simulink model "mbd_example_test"  (R2022b)
settings: Solver=FixedStepDiscrete  StartTime=0.0  StopTime=10.0  RelTol=1e-3  EnableMultiTasking=on
PostLoadFcn:
  | run([bdroot '_init']);
InitFcn:
  | checkModelFolder(true); % Optional
  | run([bdroot '_init']);
undefined symbols (not defined in the file or in its folder): MBDDiag_Comm_Module, MBDDiag_Comm_Type
libraries: MbdLib_Uart x9, MbdLib_Usb x8, MbdLib_Digital x7, MbdLib_Pwm x6, MbdLib_Qdec x6, MbdLib_Sys x5, MbdLib_LpTimer x5, MbdLib_Nvmem x5, MbdLib_Analog x4, MbdLib_Can x3, MbdLib_I2c x2, MbdLib_Ic x2
settings Model: Creator=KenYoshioka  LastModifiedBy=KenYoshioka
settings SolverCC: AutoInsertRateTranBlk=on
settings OptimizationCC: DefaultParameterBehavior=Inlined  DefaultUnderspecifiedDataType=single  EnhancedBackFolding=on  BooleansAsBitfields=on  PassReuseOutputArgsAs=Individual arguments  ZeroExternalMemoryAtStartup=off  ZeroInternalMemoryAtStartup=off  OptimizeBlockOrder=speed  DifferentSizesBufferReuse=on  EfficientTunableParamExpr=on
settings DebuggingCC: ParameterTunabilityLossMsg=error
settings HardwareCC: ProdBitPerPointer=32  ProdBitPerSizeT=32  ProdBitPerPtrDiffT=32  ProdLargestAtomicInteger=Long  ProdLargestAtomicFloat=Double  ProdWordSize=32  ProdHWDeviceType=ARM Compatible->ARM Cortex-M
settings ModelReferenceCC: EnableRefExpFcnMdlSchedulingChecks=on  ModelReferenceNumInstancesAllowed=Single
settings SFSimCC: MATLABDynamicMemAlloc=off
settings RTWCC: Description=MBD Embedded Target STM32 Cortex M4 (real-time)  SystemTargetFile=MBD_STM32_stf.tlc  TemplateMakefile=MBD_STM32.tmf  Toolchain=arm-none-eabi - v9.3.1
settings CodeAppCC: ForceParamTrailComments=on  IgnoreCustomStorageClasses=off  MaxIdLength=255  OperatorAnnotations=on  SimulinkDataObjDesc=on  SFDataObjDesc=on  InsertBlockDesc=on
settings STFCustomTargetCC: MultiwordLength=256  IncludeMdlTerminateFcn=off  CombineOutputUpdateFcns=on  CombineSignalStateStructs=on  SuppressErrorStatus=on  ERTCustomFileBanners=on  SupportContinuousTime=off  RemoveResetFunc=on  MATLABClassNameForMDSCustomization=Simulink.SoftwareTarget.ERTCustomization  UseToolchainInfoCompliant=on  SystemTargetFile=MBD_STM32_stf.tlc
settings ERTTargetCC: ParMdlRefBuildCompliant=off  CompOptLevelCompliant=off  ConcurrentExecutionCompliant=off  IncludeMdlTerminateFcn=off  CombineSignalStateStructs=on  SuppressErrorStatus=on  SupportNonInlinedSFcns=on  ModelStepFunctionPrototypeControlCompliant=off  CPPClassGenCompliant=off  ExtModeStaticAllocSize=2000  InlinedParameterPlacement=NonHierarchical  ERTCustomFileTemplate=mbd_lib_interface.tlc  MaxLineWidth=110

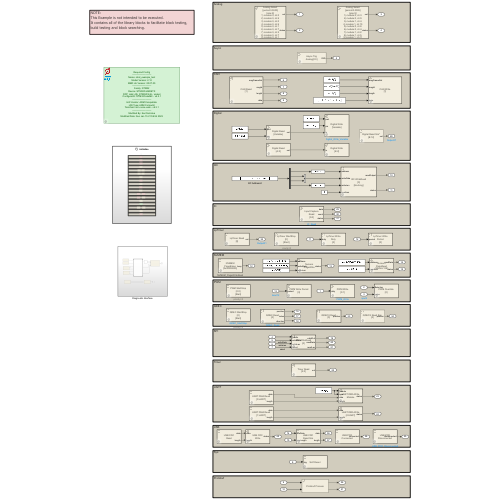
[thumbnail: Simulink's stored preview of the top-level diagram]
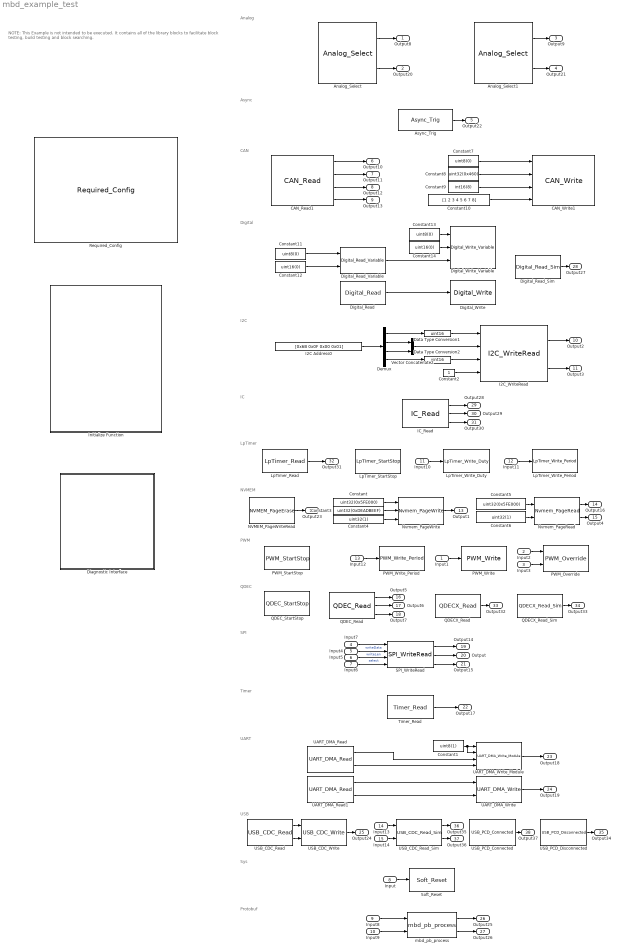
== system mbd_example_test ==
  note: NOTE:
      | This Example is not intended to be executed.
      | It contains all of the library blocks to facilitate block testing,
      | build testing and block searching.
  note: UART
  note: SPI
  note: NVMEM
  note: I2C
  note: CAN
  note: Digital
  note: QDEC
  note: PWM
  note: Analog
  note: Timer
  note: Async
  note: USB
  note: Sys
  note: Protobuf
  note: IC
  note: LpTimer
  Input1 : Inport
  Input2 : Inport  Port=2
  Input3 : Inport  Port=3
  Input7 : Inport  Port=4  OutDataTypeStr=boolean
  Input4 : Inport  Port=5  OutDataTypeStr=uint8
  Input5 : Inport  Port=6  OutDataTypeStr=uint16
  Input6 : Inport  Port=7
  Input : Inport  Port=8
  Input8 : Inport  Port=9
  Input9 : Inport  Port=10
  Input10 : Inport  Port=11
  Input11 : Inport  Port=12
  Input12 : Inport  Port=13
  Input13 : Inport  Port=14
  Input14 : Inport  Port=15
  Analog_Select : MbdLib_Analog/Analog_Select  Param_triggerMode=No trigger  Param_module=0  Param_timeout=0  Param_outputNum=9  Param_module1=0  Param_index1=0  Param_module2=0  Param_index2=1  Param_module3=0  Param_index3=2  Param_module4=0  Param_index4=3  Param_module5=0  Param_index5=4  Param_module6=0  Param_index6=5  Param_module7=0  Param_index7=6  Param_module8=0  Param_index8=7  Param_module9=0  Param_index9=8  Param_module10=0  Param_index10=9  Param_module11=0  Param_index11=10  Param_module12=0  Param_index12=11  Param_sampleTime=T_s_COMM  Param_MBDUpdate=1
      settings: SourceProductName=Peloton Interface Library
  Analog_Select1 : MbdLib_Analog/Analog_Select  Param_triggerMode=No trigger  Param_module=0  Param_timeout=0  Param_outputNum=9  Param_module1=0  Param_index1=0  Param_module2=0  Param_index2=1  Param_module3=1  Param_index3=2  Param_module4=1  Param_index4=3  Param_module5=0  Param_index5=4  Param_module6=0  Param_index6=5  Param_module7=1  Param_index7=6  Param_module8=1  Param_index8=7  Param_module9=1  Param_index9=8  Param_module10=0  Param_index10=9  Param_module11=0  Param_index11=10  Param_module12=0  Param_index12=11  Param_sampleTime=T_s_COMM  Param_MBDUpdate=1
      settings: SourceProductName=Peloton Interface Library
  Async_Trig : MbdLib_Async/Async_Trig  Param_source=Analog  Param_module=0  Param_ch=0  Param_sampleTime=-1
      settings: SourceProductName=Peloton Interface Library
  CAN_Read1 : MbdLib_Can/CAN_Read  Param_module=1  Param_sampleTime=T_s_COMM
      settings: SourceProductName=Peloton Interface Library
  CAN_Write1 : MbdLib_Can/CAN_Write  Param_module=1  Param_sampleTime=T_s_COMM
      settings: SourceProductName=Peloton Interface Library
  Constant : Constant  Value=uint32(0x5FE000)
  Constant1 : Constant  Value=uint8(1)
  Constant10 : Constant  Value=[1 2 3 4 5 6 7 8]  OutDataTypeStr=uint8
  Constant11 : Constant  Value=uint8(0)
  Constant12 : Constant  Value=uint16(0)
  Constant13 : Constant  Value=uint8(0)
  Constant14 : Constant  Value=uint16(0)
  Constant2 : Constant  OutDataTypeStr=uint16
  Constant3 : Constant  Value=uint32(0xDEADBEEF)
  Constant4 : Constant  Value=uint32(1)
  Constant5 : Constant  Value=uint32(0x5FE000)
  Constant6 : Constant  Value=uint32(1)
  Constant7 : Constant  Value=uint8(0)
  Constant8 : Constant  Value=uint32(0x460)
  Constant9 : Constant  Value=int16(8)
  Data Type Conversion1 : DataTypeConversion  OutDataTypeStr=uint16  SaturateOnIntegerOverflow=off  RndMeth=Floor
  Data Type Conversion2 : DataTypeConversion  OutDataTypeStr=uint16  SaturateOnIntegerOverflow=off  RndMeth=Floor
  Demux : Demux
  Diagnostic Interface : Subsystem
  Digital_Read : MbdLib_Digital/Digital_Read  Param_module=A  Param_ch=0  Param_sampleTime=T_s_COMM  Sim_invert=off  Sim_out=0
      settings: SourceProductName=Peloton Interface Library
  Digital_Read_Sim : MbdLib_Digital/Digital_Read_Sim  Param_module=B  Param_ch=12  Param_sampleTime=Tfast_s  Sim_invert=on  Sim_out=0  Sim_enable=on  Sim_simin=sim_knob1Button
      settings: SourceProductName=Peloton Interface Library
  Digital_Read_Variable : MbdLib_Digital/Digital_Read_Variable  Param_sampleTime=T_s_COMM  Sim_invert=off  Sim_out=0
      settings: SourceProductName=Peloton Interface Library
  Digital_Write : MbdLib_Digital/Digital_Write  Param_module=E  Param_ch=2  Param_sampleTime=-1
      settings: SourceProductName=Peloton Interface Library
  Digital_Write_Variable : MbdLib_Digital/Digital_Write_Variable  Param_sampleTime=-1
      settings: SourceProductName=Peloton Interface Library
  I2C Address0 : Constant  Value=[0x6B 0x0F 0x00 0x01]  OutDataTypeStr=uint8
  I2C_WriteRead : MbdLib_I2c/I2C_WriteRead  Param_module=0  Param_writeLim=2  Param_readLim=1  Param_mode=blocking  Param_timeout=0  Param_sampleTime=T_s_COMM
      settings: SourceProductName=Peloton Interface Library
  IC_Read : MbdLib_Ic/IC_Read  Param_module=0  Param_ch=0  Param_width=byte  Param_length=0  Param_sampleTime=-1
      settings: SourceProductName=Peloton Interface Library
  Initialize Function : Subsystem  TreatAsAtomicUnit=on
  LpTimer_Read : MbdLib_LpTimer/LpTimer_Read  Param_module=0  Param_sampleTime=-1
      settings: SourceProductName=Peloton Interface Library
  LpTimer_StartStop : MbdLib_LpTimer/LpTimer_StartStop  Priority=0  Param_module=0  Param_action=Start  Param_mode=PWM  Param_period=0  Param_duty=0  Param_priority=0  Param_sampleTime=-1
      settings: AttributesFormatString=priority=%<priority>  SourceProductName=Peloton Interface Library
  LpTimer_Write_Duty : MbdLib_LpTimer/LpTimer_Write_Duty  Param_module=0  Param_sampleTime=-1
      settings: SourceProductName=Peloton Interface Library
  LpTimer_Write_Period : MbdLib_LpTimer/LpTimer_Write_Period  Param_module=0  Param_sampleTime=-1
      settings: SourceProductName=Peloton Interface Library
  NVMEM_PageWriteRead : MbdLib_Nvmem/NVMEM_PageErase  Param_address=0  Param_sampleTime=-1
      settings: SourceProductName=Peloton Interface Library
  Nvmem_PageRead : MbdLib_Nvmem/Nvmem_PageRead  Param_wordLim=128  Param_sampleTime=T_s_COMM
      settings: SourceProductName=Peloton Interface Library
  Nvmem_PageWrite : MbdLib_Nvmem/Nvmem_PageWrite  Param_sampleTime=T_s_COMM
      settings: SourceProductName=Peloton Interface Library
  PWM_Override : MbdLib_Pwm/PWM_Override  Param_module=0  Param_sampleTime=T_s_COMM
      settings: SourceProductName=Peloton Interface Library
  PWM_StartStop : MbdLib_Pwm/PWM_StartStop  Priority=0  Param_module=0  Param_ch=0  Param_action=Start  Param_priority=0  Param_sampleTime=-1
      settings: AttributesFormatString=priority=%<priority>  SourceProductName=Peloton Interface Library
  PWM_Write : MbdLib_Pwm/PWM_Write  Priority=1  Param_module=0  Param_ch_visible=1  Param_ch=1  Param_sync=off  Param_sampleTime=T_s_COMM
      settings: SourceProductName=Peloton Interface Library
  PWM_Write_Period : MbdLib_Pwm/PWM_Write_Period  Param_module=0  Param_sampleTime=-1
      settings: SourceProductName=Peloton Interface Library
  QDECX_Read : MbdLib_Qdec/QDECX_Read  Param_module=0  Param_sampleTime=-1  Sim_position=0
      settings: SourceProductName=Peloton Interface Library
  QDECX_Read_Sim : MbdLib_Qdec/QDECX_Read_Sim  Param_module=0  Param_sampleTime=-1  Sim_position=0  Sim_enable=off  Sim_simin=mbdSim_knob1Position
      settings: SourceProductName=Peloton Interface Library
  QDEC_Read : MbdLib_Qdec/QDEC_Read  Param_module=0  Param_dirOut=off  Param_sampleTime=T_s_COMM  Sim_position=0  Sim_index=0  Sim_direction=0
      settings: SourceProductName=Peloton Interface Library
  QDEC_StartStop : MbdLib_Qdec/QDEC_StartStop  Priority=0  Param_module=0  Param_action=Start  Param_priority=0  Param_sampleTime=-1
      settings: AttributesFormatString=priority=%<priority>  SourceProductName=Peloton Interface Library
  Required_Config : MbdLib_Required/Required_Config  Tag=MBD_Target_Info  Param_update=1
      settings: SourceProductName=Peloton Interface Library
  SPI_WriteRead : MbdLib_Spi/SPI_WriteRead  Param_module=0  Param_sampleTime=T_s_COMM
      settings: SourceProductName=Peloton Interface Library
  Soft_Reset : MbdLib_Sys/Soft_Reset  Param_sampleTime=-1
      settings: SourceProductName=Peloton Interface Library
  Timer_Read : MbdLib_Timer/Timer_Read  Param_module=2  Param_ch=0  Param_sampleTime=T_s_COMM
      settings: SourceProductName=Peloton Interface Library
  UART_DMA_Read : MbdLib_Uart/UART_DMA_Read  Param_module=0  Param_type=UART  Param_readLim=1  Param_sampleTime=T_s_COMM
      settings: SourceProductName=Peloton Interface Library
  UART_DMA_Read1 : MbdLib_Uart/UART_DMA_Read  Param_module=1  Param_type=UART  Param_readLim=1  Param_sampleTime=T_s_COMM
      settings: SourceProductName=Peloton Interface Library
  UART_DMA_Write : MbdLib_Uart/UART_DMA_Write  Param_module=0  Param_type=UART  Param_sampleTime=-1  Sim_status=0
      settings: SourceProductName=Peloton Interface Library
  UART_DMA_Write_Module : MbdLib_Uart/UART_DMA_Write_Module  Param_instanceNum=1  Param_module1=0  Param_type1=UART  Param_module2=0  Param_type2=UART  Param_module3=0  Param_type3=UART  Param_module4=0  Param_type4=UART  Param_sampleTime=-1  Sim_status=0
      settings: SourceProductName=Peloton Interface Library
  USB_CDC_Read : MbdLib_Usb/USB_CDC_Read  Param_readLim=1  Param_sampleTime=-1
      settings: SourceProductName=Peloton Interface Library
  USB_CDC_Read_Sim : MbdLib_Usb/USB_CDC_Read_Sim  Param_readLim=1  Param_sampleTime=-1
      settings: SourceProductName=Peloton Interface Library
  USB_CDC_Write : MbdLib_Usb/USB_CDC_Write  Param_sampleTime=-1  Sim_status=0
      settings: SourceProductName=Peloton Interface Library
  USB_PCD_Connected : MbdLib_Usb/USB_PCD_Connected  Param_sampleTime=-1  Sim_connected=0
      settings: SourceProductName=Peloton Interface Library
  USB_PCD_Disconnected : MbdLib_Usb/USB_PCD_Disconnected  Param_sampleTime=-1  Sim_disconnected=0
      settings: SourceProductName=Peloton Interface Library
  Vector Concatenate2 : Concatenate
  mbd_pb_process : mbd_pb/mbd_pb_process  Edit_fileName=untitled  Popup_fileExt=.proto  Param_readSize=1024  Param_writeSize=1024
      settings: SourceProductName=Peloton Component Library
  Output8 : Outport
  Output20 : Outport  Port=2
  Output9 : Outport  Port=3
  Output21 : Outport  Port=4
  Output22 : Outport  Port=5
  Output10 : Outport  Port=6
  Output11 : Outport  Port=7
  Output12 : Outport  Port=8
  Output13 : Outport  Port=9
  Output2 : Outport  Port=10
  Output3 : Outport  Port=11
  Output23 : Outport  Port=12
  Output1 : Outport  Port=13
  Output16 : Outport  Port=14
  Output4 : Outport  Port=15
  Output5 : Outport  Port=16
  Output6 : Outport  Port=17
  Output7 : Outport  Port=18
  Output14 : Outport  Port=19
  Output : Outport  Port=20
  Output15 : Outport  Port=21
  Output17 : Outport  Port=22
  Output18 : Outport  Port=23
  Output19 : Outport  Port=24
  Output24 : Outport  Port=25
  Output25 : Outport  Port=26
  Output26 : Outport  Port=27
  Output27 : Outport  Port=28
  Output28 : Outport  Port=29
  Output29 : Outport  Port=30
  Output30 : Outport  Port=31
  Output31 : Outport  Port=32
  Output32 : Outport  Port=33
  Output33 : Outport  Port=34
  Output34 : Outport  Port=35
  Output35 : Outport  Port=36
  Output36 : Outport  Port=37
  Output37 : Outport  Port=38
  wires:
  Constant/1 -> Nvmem_PageWrite/1
  Input6/1 -> SPI_WriteRead/4  "select"
  Constant6/1 -> Nvmem_PageRead/2
  Constant7/1 -> CAN_Write1/1
  UART_DMA_Read1/2 -> UART_DMA_Write/2
  Input4/1 -> SPI_WriteRead/2  "writeData"
  I2C_WriteRead/1 -> Output2/1
  Analog_Select1/1 -> Output9/1
  Constant12/1 -> Digital_Read_Variable/2
  SPI_WriteRead/2 -> Output/1
  Data Type Conversion2/1 -> I2C_WriteRead/3
  Nvmem_PageRead/1 -> Output16/1
  Constant5/1 -> Nvmem_PageRead/1
  CAN_Read1/2 -> Output11/1
  QDEC_Read/3 -> Output7/1
  Constant14/1 -> Digital_Write_Variable/2
  Constant13/1 -> Digital_Write_Variable/1
  Data Type Conversion1/1 -> I2C_WriteRead/1
  UART_DMA_Write/1 -> Output19/1
  Constant1/1 -> UART_DMA_Write_Module/2, UART_DMA_Write_Module/1
  Constant8/1 -> CAN_Write1/2
  QDEC_Read/2 -> Output6/1
  Digital_Read_Variable/1 -> Digital_Write_Variable/3
  Nvmem_PageWrite/1 -> Output1/1
  Constant9/1 -> CAN_Write1/3
  Vector Concatenate2/1 -> I2C_WriteRead/2
  Constant11/1 -> Digital_Read_Variable/1
  UART_DMA_Read1/1 -> UART_DMA_Write/1
  SPI_WriteRead/1 -> Output14/1
  Demux/4 -> Data Type Conversion2/1
  CAN_Read1/4 -> Output13/1
  Input1/1 -> PWM_Write/1
  Constant3/1 -> Nvmem_PageWrite/2
  SPI_WriteRead/3 -> Output15/1
  Input3/1 -> PWM_Override/2
  Demux/2 -> Vector Concatenate2/1
  CAN_Read1/1 -> Output10/1
  Constant4/1 -> Nvmem_PageWrite/3
  I2C Address0/1 -> Demux/1
  QDEC_Read/1 -> Output5/1
  Input7/1 -> SPI_WriteRead/1
  Demux/3 -> Vector Concatenate2/2
  Timer_Read/1 -> Output17/1
  Digital_Read/1 -> Digital_Write/1
  Nvmem_PageRead/2 -> Output4/1
  I2C_WriteRead/2 -> Output3/1
  Analog_Select/1 -> Output8/1
  Input2/1 -> PWM_Override/1
  Input5/1 -> SPI_WriteRead/3  "writeLen"
  UART_DMA_Read/2 -> UART_DMA_Write_Module/4
  Constant10/1 -> CAN_Write1/4
  CAN_Read1/3 -> Output12/1
  UART_DMA_Read/1 -> UART_DMA_Write_Module/3
  UART_DMA_Write_Module/1 -> Output18/1
  Constant2/1 -> I2C_WriteRead/4
  Demux/1 -> Data Type Conversion1/1
  Analog_Select/2 -> Output20/1
  Analog_Select1/2 -> Output21/1
  Async_Trig/1 -> Output22/1
  NVMEM_PageWriteRead/1 -> Output23/1
  USB_CDC_Read/1 -> USB_CDC_Write/1
  USB_CDC_Read/2 -> USB_CDC_Write/2
  USB_CDC_Write/1 -> Output24/1
  Input/1 -> Soft_Reset/1
  Input8/1 -> mbd_pb_process/1
  Input9/1 -> mbd_pb_process/2
  mbd_pb_process/1 -> Output25/1
  mbd_pb_process/2 -> Output26/1
  Digital_Read_Sim/1 -> Output27/1
  IC_Read/1 -> Output28/1
  IC_Read/2 -> Output29/1
  IC_Read/3 -> Output30/1
  LpTimer_Read/1 -> Output31/1
  Input10/1 -> LpTimer_Write_Duty/1
  Input11/1 -> LpTimer_Write_Period/1
  Input12/1 -> PWM_Write_Period/1
  QDECX_Read/1 -> Output32/1
  QDECX_Read_Sim/1 -> Output33/1
  USB_PCD_Disconnected/1 -> Output34/1
  USB_CDC_Read_Sim/1 -> Output35/1
  USB_CDC_Read_Sim/2 -> Output36/1
  USB_PCD_Connected/1 -> Output37/1
  Input13/1 -> USB_CDC_Read_Sim/1
  Input14/1 -> USB_CDC_Read_Sim/2

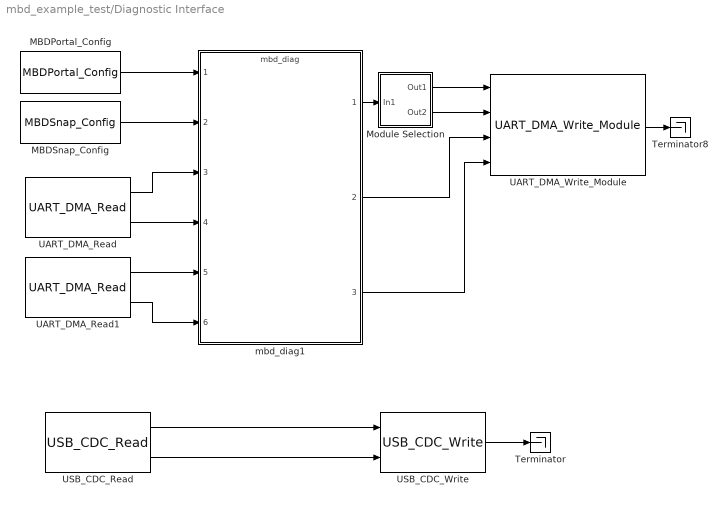
== system mbd_example_test/Diagnostic Interface ==
  MBDPortal_Config : MbdLib_PortalDiag/MBDPortal_Config  Param_SigMax=MBDPortal_SignalNum  Param_ParamMax=MBDPortal_ParamNum
      settings: SourceProductName=Peloton Component Library
  MBDSnap_Config : MbdLib_SnapDiag/MBDSnap_Config  Priority=-5000  Param_enableAll=on  Param_SampleTime=T_s_COMM  Param_SigMax=MBDSnap_SignalNum
      settings: SourceProductName=Peloton Component Library
  Module Selection : Subsystem
  Terminator : Terminator
  Terminator8 : Terminator
  UART_DMA_Read : MbdLib_Uart/UART_DMA_Read  Tag=TAG_UART_DMA  Param_module=MBDDiag_Comm_Module(1)  Param_type=USART  Param_readLim=100  Param_sampleTime=T_s_COMM
      settings: SourceProductName=Peloton Interface Library
  UART_DMA_Read1 : MbdLib_Uart/UART_DMA_Read  Tag=TAG_UART_DMA  Param_module=MBDDiag_Comm_Module(2)  Param_type=USART  Param_readLim=100  Param_sampleTime=T_s_COMM
      settings: SourceProductName=Peloton Interface Library
  UART_DMA_Write_Module : MbdLib_Uart/UART_DMA_Write_Module  Param_instanceNum=2  Param_module1=MBDDiag_Comm_Module(1)  Param_type1=USART  Param_module2=MBDDiag_Comm_Module(2)  Param_type2=USART  Param_module3=0  Param_type3=UART  Param_module4=0  Param_type4=UART  Param_sampleTime=-1  Sim_status=0
      settings: SourceProductName=Peloton Interface Library
  USB_CDC_Read : MbdLib_Usb/USB_CDC_Read  Param_readLim=1  Param_sampleTime=T_s_COMM
      settings: SourceProductName=Peloton Interface Library
  USB_CDC_Write : MbdLib_Usb/USB_CDC_Write  Param_sampleTime=-1  Sim_status=0
      settings: SourceProductName=Peloton Interface Library
  mbd_diag1 : ModelReference  ModelNameDialog=mbd_diag.slx  SimulationMode=Normal  ModelReferenceVersion=2.247  SimulationMode=Normal
  wires:
  Module Selection/2(Out2) -> UART_DMA_Write_Module/2
  UART_DMA_Read1/2 -> mbd_diag1/6
  UART_DMA_Read/1 -> mbd_diag1/3
  UART_DMA_Write_Module/1 -> Terminator8/1
  mbd_diag1/1 -> Module Selection/1(In1)
  MBDPortal_Config/1 -> mbd_diag1/1
  mbd_diag1/3 -> UART_DMA_Write_Module/4
  MBDSnap_Config/1 -> mbd_diag1/2
  mbd_diag1/2 -> UART_DMA_Write_Module/3
  UART_DMA_Read/2 -> mbd_diag1/4
  Module Selection/1(Out1) -> UART_DMA_Write_Module/1
  UART_DMA_Read1/1 -> mbd_diag1/5
  USB_CDC_Read/1 -> USB_CDC_Write/1
  USB_CDC_Read/2 -> USB_CDC_Write/2
  USB_CDC_Write/1 -> Terminator/1

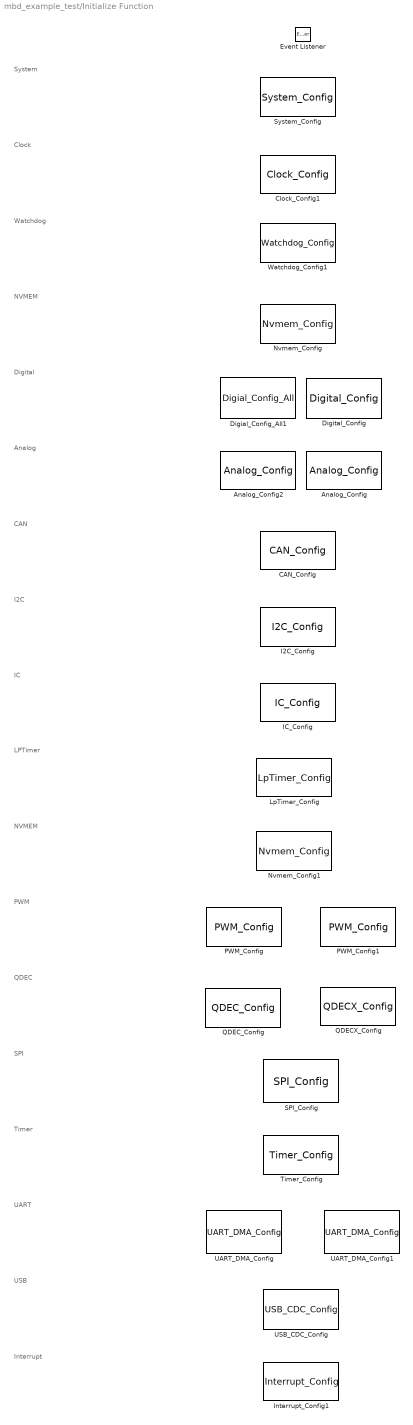
== system mbd_example_test/Initialize Function ==
  note: Analog
  note: CAN
  note: Digital
  note: I2C
  note: PWM
  note: QDEC
  note: SPI
  note: Timer
  note: UART
  note: NVMEM
  note: Clock
  note: Watchdog
  note: Interrupt
  note: System
  note: USB
  note: IC
  note: LPTimer
  note: NVMEM
  Analog_Config : MbdLib_Analog/Analog_Config  Priority=50  Param_module=1  Param_step=-1  Param_preScaler=3  Param_startUpTime=4  Param_signMode=2  Param_resolution=0  Param_hwTrigEn=on  Param_hwTrigSel=4  Param_swTrigEn=off  Param_gainEnable=on  Param_channels={ '0', 'on', 'B', '1', '0', '0', '512', 'off', 'on'; '1', 'on', 'C', '13', '1', '0', '512', 'off', 'on'; '2', 'on', 'C', '15', '3', '0', '512', 'off', 'off'; '3', 'off', 'A', '0', 'disable', '0', '0', 'off', 'off'; '4', 'on', 'C', '29', '2', '0', '512', 'off', 'on'; '5', 'on', 'C', '30', '4', '0', '512', 'off', 'on'; '6', 'on', 'C', '31', 'disable', '0', '512', 'off', 'off'; '7', 'on', 'C', '26', 'disable', '0', '512', 'off', 'off'; '8', 'off', 'A', '0', 'disable', '0', '0', 'off', 'off'; '9', 'off', 'A', '0', 'disable', '0', '0', 'off', 'off'; '10', 'on', 'E', '3', 'disable', '0', '512', 'off', 'off'; '11', 'on', 'E', '0', 'disable', '0', '512', 'off', 'off' }  Param_priority=50  Param_sampleTime=-1
      settings: AttributesFormatString=priority=%<priority>  SourceProductName=Peloton Interface Library
  Analog_Config2 : MbdLib_Analog/Analog_Config  Priority=50  Param_module=0  Param_step=-1  Param_preScaler=3  Param_startUpTime=4  Param_signMode=2  Param_resolution=0  Param_hwTrigEn=on  Param_hwTrigSel=4  Param_swTrigEn=off  Param_gainEnable=on  Param_channels={ '0', 'on', 'D', '30', '0', '0', '512', 'off', 'on'; '1', 'on', 'A', '21', '1', '0', '512', 'off', 'on'; '2', 'on', 'B', '3', '2', '0', '512', 'on', 'on'; '3', 'on', 'E', '5', '3', '0', '512', 'off', 'on'; '4', 'on', 'E', '4', '4', '0', '512', 'off', 'on'; '5', 'off', 'A', '0', 'disable', '0', '0', 'off', 'off'; '6', 'on', 'A', '17', 'disable', '0', '512', 'off', 'off'; '7', 'on', 'A', '18', 'disable', '0', '512', 'off', 'off'; '8', 'on', 'A', '19', 'disable', '0', '512', 'off', 'off'; '9', 'on', 'A', '20', 'disable', '0', '512', 'off', 'off'; '10', 'on', 'B', '0', 'disable', '0', '512', 'off', 'off'; '11', 'off', 'A', '0', 'disable', '0', '0', 'off', 'off' }  Param_priority=50  Param_sampleTime=-1
      settings: AttributesFormatString=priority=%<priority>  SourceProductName=Peloton Interface Library
  CAN_Config : MbdLib_Can/CAN_Config  Priority=60  Param_module=1  Param_priority=60  Param_sampleTime=-1
      settings: AttributesFormatString=priority=%<priority>  SourceProductName=Peloton Interface Library
  Clock_Config1 : MbdLib_Sys/Clock_Config  Priority=10  Param_frequency=150000000  Param_priority=10  Param_sampleTime=-1
      settings: AttributesFormatString=priority=%<priority>  SourceProductName=Peloton Interface Library
  Digial_Config_All1 : MbdLib_Digital/Digial_Config_All  Priority=40  Param_channels={ 'A', '0', 'off', '0 : input', '0 : low', '0 : none', '0 : none', '0 : low', '0 : low'; 'A', '1', 'off', '0 : input', '0 : low', '0 : none', '0 : none', '0 : low', '0 : low'; 'A', '2', 'off', '0 : input', '0 : low', '0 : none', '0 : none', '0 : low', '0 : low'; 'A', '3', 'off', '0 : input', '0 : low', '0 : none', '0 : none', '0 : low', '0 : low'; 'A', '4', 'off', '0 : input', '0 : low', '0 : none', '0 : none', '0 : low', '0 : low'; 'A', '5', 'off', '0 : input', '0 : low', '0 : none', '0 : none', '0 : low', '0 : low'; 'A', '6', 'off', '0 : input', '0 : low', '0 : none', '0 : none', '0 : low', '0 : low'; 'A', '7', 'off', '0 : input', '0 : low', '0 : none', '0 : none', '0 : low', '0 : low'; 'A', '8', 'off', '0 : input', '0 : low', '0 : none', '0 : none', '0 : low', '0 : low'; 'A', '9', 'off', '0 : input', '0 : low', '0 : none', '0 : none', '0 : low', '0 : low'; 'A', '10', 'off', '0 : input', '0 : low', '0 : none', '0 : none', '0 : low', '0 : low'; 'A', '11', 'off', '0 : input', '0 : low', '0 : none', '0 : none', '0 : low', '0 : low'; 'A', '12', 'off', '0 : input', '0 : low', '0 : none', '0 : none', '0 : low', '0 : low'; 'A', '13', 'off', '0 : input', '0 : low', '0 : none', '0 : none', '0 : low', '0 : low'; 'A', '14', 'off', '0 : input', '0 : low', '0 : none', '0 : none', '0 : low', '0 : low'; 'A', '15', 'off', '0 : input', '0 : low', '0 : none', '0 : none', '0 : low', '0 : low'; 'A', '16', 'off', '0 : input', '0 : low', '0 : none', '0 : none', '0 : low', '0 : low'; 'A', '17', 'off', '0 : input', '0 : low', '0 : none', '0 : none', '0 : low', '0 : low'; 'A', '18', 'off', '0 : input', '0 : low', '0 : none', '0 : none', '0 : low', '0 : low'; 'A', '19', 'off', '0 : input', '0 : low', '0 : none', '0 : none', '0 : low', '0 : low'; 'A', '20', 'off', '0 : input', '0 : low', '0 : none', '0 : none', '0 : low', '0 : low'; 'A', '21', 'off', '0 : input', '0 : low', '0 : none', '0 : none', '0 : low', '0 : low'; 'A', '22', 'off', '0 : input', '0 : low', '0 : none', '0 : none', '0 : low', '0 : low'; 'A', '23', 'off', '0 : input', '0 : low', '0 : none', '0 : none', '0 : low', '0 : low'; 'A', '24', 'off', '0 : input', '0 : low', '0 : none', '0 : none', '0 : low', '0 : low'; 'A', '25', 'off', '0 : input', '0 : low', '0 : none', '0 : none', '0 : low', '0 : low'; 'A', '26', 'off', '0 : input', '0 : low', '0 : none', '0 : none', '0 : low', '0 : low'; 'A', '27', 'off', '0 : input', '0 : low', '0 : none', '0 : none', '0 : low', '0 : low'; 'A', '28', 'off', '0 : input', '0 : low', '0 : none', '0 : none', '0 : low', '0 : low'; 'A', '29', 'off', '0 : input', '0 : low', '0 : none', '0 : none', '0 : low', '0 : low'; 'A', '30', 'off', '0 : input', '0 : low', '0 : none', '0 : none', '0 : low', '0 : low'; 'A', '31', 'off', '0 : input', '0 : low', '0 : none', '0 : none', '0 : low', '0 : low'; 'B', '0', 'off', '0 : input', '0 : low', '0 : none', '0 : none', '0 : low', '0 : low'; 'B', '1', 'off', '0 : input', '0 : low', '0 : none', '0 : none', '0 : low', '0 : low'; 'B', '2', 'off', '0 : input', '0 : low', '0 : none', '0 : none', '0 : low', '0 : low'; 'B', '3', 'off', '0 : input', '0 : low', '0 : none', '0 : none', '0 : low', '0 : low'; 'B', '4', 'off', '0 : input', '0 : low', '0 : none', '0 : none', '0 : low', '0 : low'; 'B', '5', 'off', '0 : input', '0 : low', '0 : none', '0 : none', '0 : low', '0 : low'; 'B', '6', 'off', '0 : input', '0 : low', '0 : none', '0 : none', '0 : low', '0 : low'; 'B', '7', 'off', '0 : input', '0 : low', '0 : none', '0 : none', '0 : low', '0 : low'; 'B', '8', 'off', '0 : input', '0 : low', '0 : none', '0 : none', '0 : low', '0 : low'; 'B', '9', 'off', '0 : input', '0 : low', '0 : none', '0 : none', '0 : low', '0 : low'; 'B', '10', 'off', '0 : input', '0 : low', '0 : none', '0 : none', '0 : low', '0 : low'; 'B', '11', 'off', '0 : input', '0 : low', '0 : none', '0 : none', '0 : low', '0 : low'; 'B', '12', 'off', '0 : input', '0 : low', '0 : none', '0 : none', '0 : low', '0 : low'; 'B', '13', 'off', '0 : input', '0 : low', '0 : none', '0 : none', '0 : low', '0 : low'; 'C', '0', 'off', '0 : input', '0 : low', '0 : none', '0 : none', '0 : low', '0 : low'; 'C', '1', 'off', '0 : input', '0 : low', '0 : none', '0 : none', '0 : low', '0 : low'; 'C', '2', 'off', '0 : input', '0 : low', '0 : none', '0 : none', '0 : low', '0 : low'; 'C', '3', 'off', '0 : input', '0 : low', '0 : none', '0 : none', '0 : low', '0 : low'; 'C', '4', 'off', '0 : input', '0 : low', '0 : none', '0 : none', '0 : low', '0 : low'; 'C', '5', 'off', '0 : input', '0 : low', '0 : none', '0 : none', '0 : low', '0 : low'; 'C', '6', 'off', '0 : input', '0 : low', '0 : none', '0 : none', '0 : low', '0 : low'; 'C', '7', 'off', '0 : input', '0 : low', '0 : none', '0 : none', '0 : low', '0 : low'; 'C', '8', 'off', '0 : input', '0 : low', '0 : none', '0 : none', '0 : low', '0 : low'; 'C', '9', 'off', '0 : input', '0 : low', '0 : none', '0 : none', '0 : low', '0 : low'; 'C', '10', 'off', '0 : input', '0 : low', '0 : none', '0 : none', '0 : low', '0 : low'; 'C', '11', 'off', '0 : input', '0 : low', '0 : none', '0 : none', '0 : low', '0 : low'; 'C', '12', 'off', '0 : input', '0 : low', '0 : none', '0 : none', '0 : low', '0 : low'; 'C', '13', 'off', '0 : input', '0 : low', '0 : none', '0 : none', '0 : low', '0 : low'; 'C', '14', 'off', '0 : input', '0 : low', '0 : none', '0 : none', '0 : low', '0 : low'; 'C', '15', 'off', '0 : input', '0 : low', '0 : none', '0 : none', '0 : low', '0 : low'; 'C', '16', 'off', '0 : input', '0 : low', '0 : none', '0 : none', '0 : low', '0 : low'; 'C', '17', 'off', '0 : input', '0 : low', '0 : none', '0 : none', '0 : low', '0 : low'; 'C', '18', 'off', '0 : input', '0 : low', '0 : none', '0 : none', '0 : low', '0 : low'; 'C', '19', 'off', '0 : input', '0 : low', '0 : none', '0 : none', '0 : low', '0 : low'; 'C', '20', 'off', '0 : input', '0 : low', '0 : none', '0 : none', '0 : low', '0 : low'; 'C', '21', 'off', '0 : input', '0 : low', '0 : none', '0 : none', '0 : low', '0 : low'; 'C', '22', 'off', '0 : input', '0 : low', '0 : none', '0 : none', '0 : low', '0 : low'; 'C', '23', 'off', '0 : input', '0 : low', '0 : none', '0 : none', '0 : low', '0 : low'; 'C', '24', 'off', '0 : input', '0 : low', '0 : none', '0 : none', '0 : low', '0 : low'; 'C', '25', 'off', '0 : input', '0 : low', '0 : none', '0 : none', '0 : low', '0 : low'; 'C', '26', 'off', '0 : input', '0 : low', '0 : none', '0 : none', '0 : low', '0 : low'; 'C', '27', 'off', '0 : input', '0 : low', '0 : none', '0 : none', '0 : low', '0 : low'; 'C', '28', 'off', '0 : input', '0 : low', '0 : none', '0 : none', '0 : low', '0 : low'; 'C', '29', 'off', '0 : input', '0 : low', '0 : none', '0 : none', '0 : low', '0 : low'; 'C', '30', 'off', '0 : input', '0 : low', '0 : none', '0 : none', '0 : low', '0 : low'; 'C', '31', 'off', '0 : input', '0 : low', '0 : none', '0 : none', '0 : low', '0 : low'; 'D', '0', 'off', '0 : input', '0 : low', '0 : none', '0 : none', '0 : low', '0 : low'; 'D', '1', 'off', '0 : input', '0 : low', '0 : none', '0 : none', '0 : low', '0 : low'; 'D', '2', 'off', '0 : input', '0 : low', '0 : none', '0 : none', '0 : low', '0 : low'; 'D', '3', 'off', '0 : input', '0 : low', '0 : none', '0 : none', '0 : low', '0 : low'; 'D', '4', 'off', '0 : input', '0 : low', '0 : none', '0 : none', '0 : low', '0 : low'; 'D', '5', 'off', '0 : input', '0 : low', '0 : none', '0 : none', '0 : low', '0 : low'; 'D', '6', 'off', '0 : input', '0 : low', '0 : none', '0 : none', '0 : low', '0 : low'; 'D', '7', 'off', '0 : input', '0 : low', '0 : none', '0 : none', '0 : low', '0 : low'; 'D', '8', 'off', '0 : input', '0 : low', '0 : none', '0 : none', '0 : low', '0 : low'; 'D', '9', 'off', '0 : input', '0 : low', '0 : none', '0 : none', '0 : low', '0 : low'; 'D', '10', 'off', '0 : input', '0 : low', '0 : none', '0 : none', '0 : low', '0 : low'; 'D', '11', 'off', '0 : input', '0 : low', '0 : none', '0 : none', '0 : low', '0 : low'; 'D', '12', 'off', '0 : input', '0 : low', '0 : none', '0 : none', '0 : low', '0 : low'; 'D', '13', 'off', '0 : input', '0 : low', '0 : none', '0 : none', '0 : low', '0 : low'; 'D', '14', 'off', '0 : input', '0 : low', '0 : none', '0 : none', '0 : low', '0 : low'; 'D', '15', 'off', '0 : input', '0 : low', '0 : none', '0 : none', '0 : low', '0 : low'; 'D', '16', 'off', '0 : input', '0 : low', '0 : none', '0 : none', '0 : low', '0 : low'; 'D', '17', 'off', '0 : input', '0 : low', '0 : none', '0 : none', '0 : low', '0 : low'; 'D', '18', 'off', '0 : input', '0 : low', '0 : none', '0 : none', '0 : low', '0 : low'; 'D', '19', 'off', '0 : input', '0 : low', '0 : none', '0 : none', '0 : low', '0 : low'; 'D', '20', 'off', '0 : input', '0 : low', '0 : none', '0 : none', '0 : low', '0 : low'; 'D', '21', 'off', '0 : input', '0 : low', '0 : none', '0 : none', '0 : low', '0 : low'; 'D', '22', 'off', '0 : input', '0 : low', '0 : none', '0 : none', '0 : low', '0 : low'; 'D', '23', 'off', '0 : input', '0 : low', '0 : none', '0 : none', '0 : low', '0 : low'; 'D', '24', 'off', '0 : input', '0 : low', '0 : none', '0 : none', '0 : low', '0 : low'; 'D', '25', 'off', '0 : input', '0 : low', '0 : none', '0 : none', '0 : low', '0 : low'; 'D', '26', 'off', '0 : input', '0 : low', '0 : none', '0 : none', '0 : low', '0 : low'; 'D', '27', 'off', '0 : input', '0 : low', '0 : none', '0 : none', '0 : low', '0 : low'; 'D', '28', 'off', '0 : input', '0 : low', '0 : none', '0 : none', '0 : low', '0 : low'; 'D', '29', 'off', '0 : input', '0 : low', '0 : none', '0 : none', '0 : low', '0 : low'; 'D', '30', 'off', '0 : input', '0 : low', '0 : none', '0 : none', '0 : low', '0 : low'; 'D', '31', 'off', '0 : input', '0 : low', '0 : none', '0 : none', '0 : low', '0 : low'; 'E', '0', 'off', '0 : input', '0 : low', '0 : none', '0 : none', '0 : low', '0 : low'; 'E', '1', 'off', '0 : input', '0 : low', '0 : none', '0 : none', '0 : low', '0 : low'; 'E', '2', 'off', '0 : input', '0 : low', '0 : none', '0 : none', '0 : low', '0 : low'; 'E', '3', 'off', '0 : input', '0 : low', '0 : none', '0 : none', '0 : low', '0 : low'; 'E', '4', 'off', '0 : input', '0 : low', '0 : none', '0 : none', '0 : low', '0 : low'; 'E', '5', 'off', '0 : input', '0 : low', '0 : none', '0 : none', '0 : low', '0 : low' }  Param_priority=40  Param_sampleTime=-1
      settings: AttributesFormatString=priority=%<priority>  SourceProductName=Peloton Interface Library
  Digital_Config : MbdLib_Digital/Digital_Config  Priority=40  Param_module=A  Param_ch=0  Param_dir=input  Param_pupd=none  Param_default=low  Param_mode=none  Param_drive=low  Param_speed=low  Param_priority=40  Param_sampleTime=-1
      settings: AttributesFormatString=priority=%<priority>  SourceProductName=Peloton Interface Library
  Event Listener : EventListener  DisableCoverage=on  EventName=reset
  I2C_Config : MbdLib_I2c/I2C_Config  Priority=70  Param_module=0  Param_priority=70  Param_sampleTime=-1
      settings: AttributesFormatString=priority=%<priority>  SourceProductName=Peloton Interface Library
  IC_Config : MbdLib_Ic/IC_Config  Priority=0  Param_module=0  Param_ch=0  Param_width=byte  Param_length=0  Param_priority=0  Param_sampleTime=-1
      settings: AttributesFormatString=priority=%<priority>  SourceProductName=Peloton Interface Library
  Interrupt_Config1 : MbdLib_Sys/Interrupt_Config  Priority=140  Param_priority=140  Param_sampleTime=-1
      settings: AttributesFormatString=priority=%<priority>  SourceProductName=Peloton Interface Library
  LpTimer_Config : MbdLib_LpTimer/LpTimer_Config  Priority=0  Param_module=0  Param_priority=0  Param_sampleTime=-1
      settings: AttributesFormatString=priority=%<priority>  SourceProductName=Peloton Interface Library
  Nvmem_Config : MbdLib_Nvmem/Nvmem_Config  Priority=30  Param_priority=30  Param_sampleTime=-1
      settings: AttributesFormatString=priority=%<priority>  SourceProductName=Peloton Interface Library
  Nvmem_Config1 : MbdLib_Nvmem/Nvmem_Config  Priority=0  Param_priority=0  Param_sampleTime=-1
      settings: AttributesFormatString=priority=%<priority>  SourceProductName=Peloton Interface Library
  PWM_Config : MbdLib_Pwm/PWM_Config  Priority=80  Param_module=0  Param_clksrc=0  Param_period=3125  Param_channels={ '0', 'on', '1563', '120', 'on'; '1', 'on', '1563', '120', 'on'; '2', 'on', '1563', '120', 'on'; '3', 'off', '0', '0', 'off' }  Param_priority=80  Param_sampleTime=-1
      settings: AttributesFormatString=priority=%<priority>  SourceProductName=Peloton Interface Library
  PWM_Config1 : MbdLib_Pwm/PWM_Config  Priority=80  Param_module=1  Param_clksrc=0  Param_period=3125  Param_channels={ '0', 'on', '1563', '120', 'on'; '1', 'on', '1563', '120', 'on'; '2', 'on', '1563', '120', 'on'; '3', 'on', '1563', '120', 'off' }  Param_priority=80  Param_sampleTime=-1
      settings: AttributesFormatString=priority=%<priority>  SourceProductName=Peloton Interface Library
  QDECX_Config : MbdLib_Qdec/QDECX_Config  Priority=0  Param_module=1  Param_portA=A  Param_pinA=0  Param_portB=A  Param_pinB=0  Param_priority=0  Param_sampleTime=-1
      settings: AttributesFormatString=priority=%<priority>  SourceProductName=Peloton Interface Library
  QDEC_Config : MbdLib_Qdec/QDEC_Config  Priority=90  Param_module=0  Param_priority=90  Param_sampleTime=-1
      settings: AttributesFormatString=priority=%<priority>  SourceProductName=Peloton Interface Library
  SPI_Config : MbdLib_Spi/SPI_Config  Priority=100  Param_module=0  Param_deviceNum=2  Param_mode1=CPOL_0_CPHA_1  Param_speed1=1Mbps  Param_select1=CS_0  Param_pin1=34  Param_mode2=CPOL_0_CPHA_1  Param_speed2=1Mbps  Param_select2=CS_1  Param_pin2=31  Param_mode3=CPOL_0_CPHA_0  Param_speed3=1Mbps  Param_select3=CS_0  Param_pin3=0  Param_mode4=CPOL_0_CPHA_0  Param_speed4=1Mbps  Param_select4=CS_0  Param_pin4=0  Param_priority=100  Param_sampleTime=-1
      settings: AttributesFormatString=priority=%<priority>  SourceProductName=Peloton Interface Library
  System_Config : MbdLib_Sys/System_Config  Priority=0  Param_priority=0  Param_sampleTime=-1
      settings: AttributesFormatString=priority=%<priority>  SourceProductName=Peloton Interface Library
  Timer_Config : MbdLib_Timer/Timer_Config  Priority=110  Param_update=1  Param_module=2  Param_step=1  Param_period=62500  Param_divider=0  Param_step0=1  Param_clksrc0=1  Param_period0=62500  Param_divider0=0  Param_step1=2  Param_clksrc1=2  Param_period1=13333  Param_divider1=0  Param_step2=3  Param_clksrc2=2  Param_period2=26666  Param_divider2=0  Param_priority=110  Param_sampleTime=-1
      settings: AttributesFormatString=priority=%<priority>  SourceProductName=Peloton Interface Library
  UART_DMA_Config : MbdLib_Uart/UART_DMA_Config  Priority=120  Param_module=0  Param_type=UART  Param_speed=921600  Param_dataBits=8  Param_stopBits=0.5  Param_parity=None  Param_priority=120  Param_sampleTime=-1
      settings: AttributesFormatString=priority=%<priority>  SourceProductName=Peloton Interface Library
  UART_DMA_Config1 : MbdLib_Uart/UART_DMA_Config  Priority=120  Param_module=1  Param_type=UART  Param_speed=921600  Param_dataBits=8  Param_stopBits=0.5  Param_parity=None  Param_priority=120  Param_sampleTime=-1
      settings: AttributesFormatString=priority=%<priority>  SourceProductName=Peloton Interface Library
  USB_CDC_Config : MbdLib_Usb/USB_CDC_Config  Priority=130  Param_bitrate=921600  Param_databits=8  Param_parity=None  Param_stopbits=1  Param_priority=130  Param_sampleTime=-1
      settings: AttributesFormatString=priority=%<priority>  SourceProductName=Peloton Interface Library
  Watchdog_Config1 : MbdLib_Sys/Watchdog_Config  Priority=20  Param_enable=off  Param_priority=20  Param_sampleTime=-1
      settings: AttributesFormatString=priority=%<priority>  SourceProductName=Peloton Interface Library

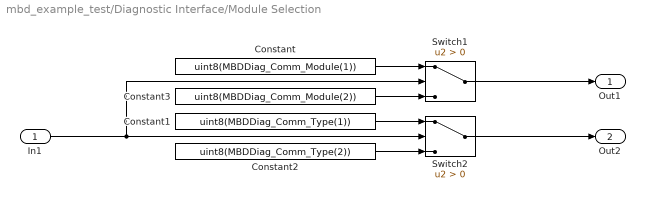
== system mbd_example_test/Diagnostic Interface/Module Selection ==
  In1 : Inport
  Constant : Constant  Value=uint8(MBDDiag_Comm_Module(1))
  Constant1 : Constant  Value=uint8(MBDDiag_Comm_Type(1))
  Constant2 : Constant  Value=uint8(MBDDiag_Comm_Type(2))
  Constant3 : Constant  Value=uint8(MBDDiag_Comm_Module(2))
  Switch1 : Switch  Criteria=u2 > Threshold  SaturateOnIntegerOverflow=off  InputSameDT=off
  Switch2 : Switch  Criteria=u2 > Threshold  SaturateOnIntegerOverflow=off  InputSameDT=off
  Out1 : Outport
  Out2 : Outport  Port=2
  wires:
  In1/1 -> Switch1/2, Switch2/2
  Constant3/1 -> Switch1/3
  Switch1/1 -> Out1/1
  Constant/1 -> Switch1/1
  Constant1/1 -> Switch2/1
  Switch2/1 -> Out2/1
  Constant2/1 -> Switch2/3
